simulink model "launcher_dir"  (R2020a)
settings: Solver=ode45  StartTime=0.0  StopTime=10.0  RelTol=1e-3
settings Model: Creator=hlf  LastModifiedBy=Aaron
settings DataIOCC: LimitDataPoints=on  SaveFormat=Array  ReturnWorkspaceOutputs=off
settings OptimizationCC: BlockReduction=off  BooleanDataType=off  LifeSpan=inf
settings DebuggingCC: SaveWithParameterizedLinksMsg=none  UnderspecifiedInitializationDetection=Classic  MergeDetectMultiDrivingBlocksExec=none  SignalResolutionControl=TryResolveAllWithWarning  SFUnexpectedBacktrackingDiag=warning  SFNoUnconditionalDefaultTransitionDiag=warning  SFExecutionAtInitializationDiag=none  ArithmeticOperatorsInVariantConditions=warning
settings HardwareCC: ProdBitPerPointer=32  ProdBitPerSizeT=32  ProdBitPerPtrDiffT=32  ProdLargestAtomicFloat=None  ProdIntDivRoundTo=Undefined  ProdEndianess=Unspecified  ProdWordSize=32  ProdHWDeviceType=32-bit Generic  TargetUnknown=on
settings ModelReferenceCC: PropagateSignalLabelsOutOfModel=off
settings SFSimCC: SimUseLocalCustomCode=off  CustomCodeUndefinedFunction=UseInterfaceOnly
settings RTWCC: RTWUseLocalCustomCode=off
settings CodeAppCC: StateflowObjectComments=on
settings GRTTargetCC: TargetLangStandard=C89/C90 (ANSI)
settings ConfigComp: CovMetricSettings=dw  CovHtmlReporting=on  CovSaveCumulativeToWorkspaceVar=on  CovSaveSingleToWorkspaceVar=on  CovExternalEMLEnable=off  CovSFcnEnable=off

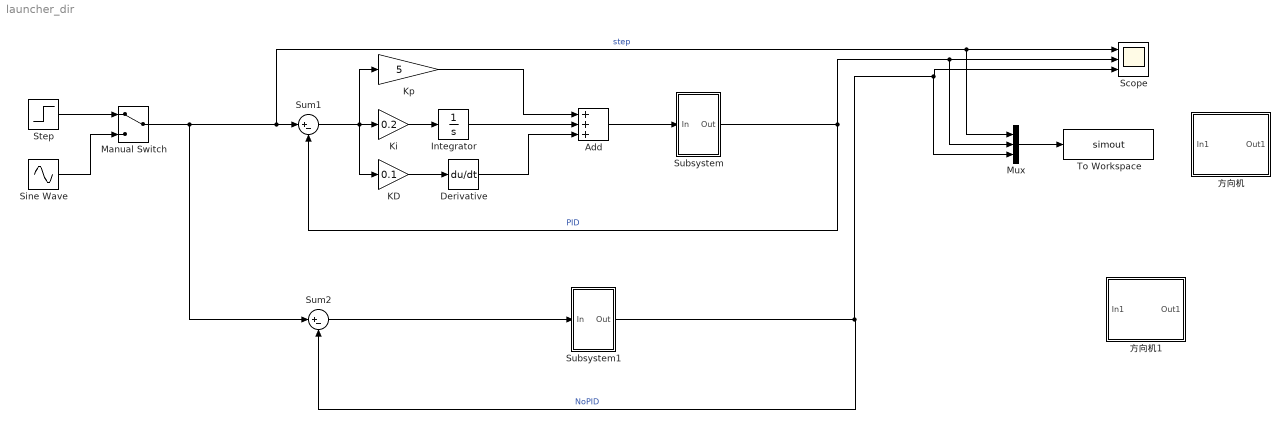
== system launcher_dir ==
  Add : Sum  Inputs=+++
  Derivative : Derivative
  Integrator : Integrator
  KD : Gain  Gain=0.1
  "Ki " : Gain  Gain=0.2
  Kp : Gain  Gain=5
  Manual Switch : ManualSwitch
  Mux : Mux  Inputs=3
  Scope : Scope  NumInputPorts=3
  Sine Wave : Sin  Frequency=2  SampleTime=0
  Step : Step  Time=0  SampleTime=0
  Subsystem : Subsystem  mask{Ka=0.004, Kf=0.25, Vm=10e-6, Dm=1.75e-5, Kq=0.043, betae=7e8, Kce=3e-13, Jt=0.0167, omegah=227, zeta=0.12}
  Subsystem1 : Subsystem  mask{Ka=0.004, Kf=0.25, Vm=10e-6, Dm=1.75e-5, Kq=0.043, betae=7e8, Kce=3e-13, Jt=0.0167, omegah=227, zeta=0.12}
  Sum1 : Sum  Inputs=|+-
  Sum2 : Sum  Inputs=|+-
  To Workspace : ToWorkspace  VariableName=simout  SaveFormat=Timeseries  SampleTime=-1
  方向机 : Subsystem
  方向机1 : Subsystem
  wires:
  Subsystem/1(Out) -> Sum1/2, Mux/2, Scope/2  "PID"
  Sum1/1 -> KD/1, Kp/1, "Ki "/1
  Manual Switch/1 -> Sum2/1, Mux/1, Scope/1, Sum1/1  "step"
  Step/1 -> Manual Switch/1
  Sine Wave/1 -> Manual Switch/2
  "Ki "/1 -> Integrator/1
  KD/1 -> Derivative/1
  Integrator/1 -> Add/2
  Kp/1 -> Add/1
  Derivative/1 -> Add/3
  Add/1 -> Subsystem/1(In)
  Subsystem1/1(Out) -> Mux/3, Scope/3, Sum2/2  "NoPID"
  Sum2/1 -> Subsystem1/1(In)
  Mux/1 -> To Workspace/1

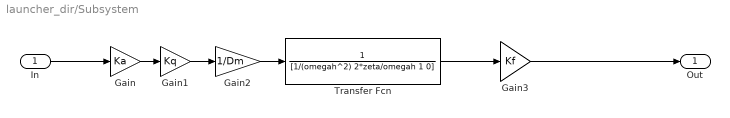
== system launcher_dir/Subsystem ==
  In : Inport
  Gain : Gain  Gain=Ka
  Gain1 : Gain  Gain=Kq
  Gain2 : Gain  Gain=1/Dm
  Gain3 : Gain  Gain=Kf
  Transfer Fcn : TransferFcn  Denominator=[1/(omegah^2) 2*zeta/omegah 1 0]
  Out : Outport
  wires:
  Gain1/1 -> Gain2/1
  Gain/1 -> Gain1/1
  In/1 -> Gain/1
  Gain2/1 -> Transfer Fcn/1
  Transfer Fcn/1 -> Gain3/1
  Gain3/1 -> Out/1

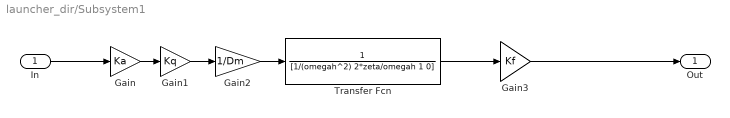
== system launcher_dir/Subsystem1 ==
  In : Inport
  Gain : Gain  Gain=Ka
  Gain1 : Gain  Gain=Kq
  Gain2 : Gain  Gain=1/Dm
  Gain3 : Gain  Gain=Kf
  Transfer Fcn : TransferFcn  Denominator=[1/(omegah^2) 2*zeta/omegah 1 0]
  Out : Outport
  wires:
  Gain1/1 -> Gain2/1
  Gain/1 -> Gain1/1
  In/1 -> Gain/1
  Gain2/1 -> Transfer Fcn/1
  Transfer Fcn/1 -> Gain3/1
  Gain3/1 -> Out/1

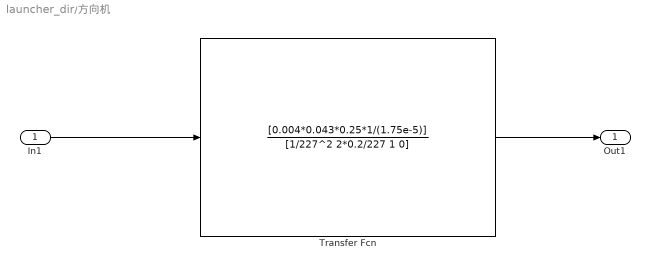
== system launcher_dir/方向机 ==
  In1 : Inport
  Transfer Fcn : TransferFcn  Numerator=[0.004*0.043*0.25*1/(1.75e-5)]  Denominator=[1/227^2 2*0.2/227 1 0]
  Out1 : Outport
  wires:
  Transfer Fcn/1 -> Out1/1
  In1/1 -> Transfer Fcn/1

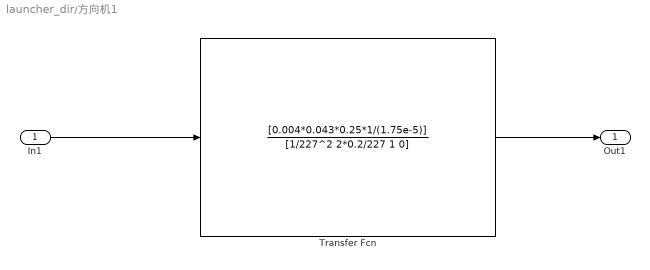
== system launcher_dir/方向机1 ==
  In1 : Inport
  Transfer Fcn : TransferFcn  Numerator=[0.004*0.043*0.25*1/(1.75e-5)]  Denominator=[1/227^2 2*0.2/227 1 0]
  Out1 : Outport
  wires:
  In1/1 -> Transfer Fcn/1
  Transfer Fcn/1 -> Out1/1
